simulink model "model"  (R2024a)
settings: Solver=VariableStepAuto  StartTime=0.0  StopTime=10  MaxStep=0.01  RelTol=1e-2
values from neighbouring files (symbols this model uses):
  K = lqr(A,B,Q,R)    [lqr_by_leg.m]    (also in setup.m = lqr_by_leg(0.218))
  N = NM + mp*diff(x + L*sin(theta),t,2)    [lqr_by_leg.m]
  T_max = 10    [setup.m]
  Tp_max = 100    [setup.m]
undefined symbols (not defined in the file or in its folder): X, Y, Z
libraries: sm_lib x86, nesl_utility x22, slpidlib x8
(part 4 of 4)

== matlab function model/forward_kinematics_virtual_speed1 ==
  data: d_phi0 output; phi_1 input; phi_4 input; d_phi1 input; d_phi4 input
function d_phi0 = fcn(phi_1,phi_4,d_phi1,d_phi4)
    L1 = 0.16;
    L2 = 0.196;
    L3 = 0.1959;
    L4 = 0.16;
    L5 = 0;
    
    d_phi0 = (d_phi1*((L1*cos(phi_1) + (2*L2*cos(2*atan(((4*L2^2*(L1*sin(phi_1) - L4*sin(phi_4))^2 - ((L1*sin(phi_1) - L4*sin(phi_4))^2 + (L5 - L1*cos(phi_1) + L4*cos(phi_4))^2 + L2^2 - L3^2)^2 + 4*L2^2*(L5 - L1*cos(phi_1) + L4*cos(phi_4))^2)^(1/2) - 2*L2*(L1*sin(phi_1) - L4*sin(phi_4)))/((L1*sin(phi_1) - L4*sin(phi_4))^2 + (L5 - L1*cos(phi_1) + L4*cos(phi_4))^2 + L2^2 - L3^2 + 2*L2*(L5 - L1*cos(phi_1) + L4*cos(phi_4)))))*(((8*L1*L2^2*cos(phi_1)*(L1*sin(phi_1) - L4*sin(phi_4)) - 2*(2*L1*cos(phi_1)*(L1*sin(phi_1) - L4*sin(phi_4)) + 2*L1*sin(phi_1)*(L5 - L1*cos(phi_1) + L4*cos(phi_4)))*((L1*sin(phi_1) - L4*sin(phi_4))^2 + (L5 - L1*cos(phi_1) + L4*cos(phi_4))^2 + L2^2 - L3^2) + 8*L1*L2^2*sin(phi_1)*(L5 - L1*cos(phi_1) + L4*cos(phi_4)))/(2*(4*L2^2*(L1*sin(phi_1) - L4*sin(phi_4))^2 - ((L1*sin(phi_1) - L4*sin(phi_4))^2 + (L5 - L1*cos(phi_1) + L4*cos(phi_4))^2 + L2^2 - L3^2)^2 + 4*L2^2*(L5 - L1*cos(phi_1) + L4*cos(phi_4))^2)^(1/2)) - 2*L1*L2*cos(phi_1))/((L1*sin(phi_1) - L4*sin(phi_4))^2 + (L5 - L1*cos(phi_1) + L4*cos(phi_4))^2 + L2^2 - L3^2 + 2*L2*(L5 - L1*cos(phi_1) + L4*cos(phi_4))) - (((4*L2^2*(L1*sin(phi_1) - L4*sin(phi_4))^2 - ((L1*sin(phi_1) - L4*sin(phi_4))^2 + (L5 - L1*cos(phi_1) + L4*cos(phi_4))^2 + L2^2 - L3^2)^2 + 4*L2^2*(L5 - L1*cos(phi_1) + L4*cos(phi_4))^2)^(1/2) - 2*L2*(L1*sin(phi_1) - L4*sin(phi_4)))*(2*L1*L2*sin(phi_1) + 2*L1*cos(phi_1)*(L1*sin(phi_1) - L4*sin(phi_4)) + 2*L1*sin(phi_1)*(L5 - L1*cos(phi_1) + L4*cos(phi_4))))/((L1*sin(phi_1) - L4*sin(phi_4))^2 + (L5 - L1*cos(phi_1) + L4*cos(phi_4))^2 + L2^2 - L3^2 + 2*L2*(L5 - L1*cos(phi_1) + L4*cos(phi_4)))^2))/(((4*L2^2*(L1*sin(phi_1) - L4*sin(phi_4))^2 - ((L1*sin(phi_1) - L4*sin(phi_4))^2 + (L5 - L1*cos(phi_1) + L4*cos(phi_4))^2 + L2^2 - L3^2)^2 + 4*L2^2*(L5 - L1*cos(phi_1) + L4*cos(phi_4))^2)^(1/2) - 2*L2*(L1*sin(phi_1) - L4*sin(phi_4)))^2/((L1*sin(phi_1) - L4*sin(phi_4))^2 + (L5 - L1*cos(phi_1) + L4*cos(phi_4))^2 + L2^2 - L3^2 + 2*L2*(L5 - L1*cos(phi_1) + L4*cos(phi_4)))^2 + 1))/(L2*cos(2*atan(((4*L2^2*(L1*sin(phi_1) - L4*sin(phi_4))^2 - ((L1*sin(phi_1) - L4*sin(phi_4))^2 + (L5 - L1*cos(phi_1) + L4*cos(phi_4))^2 + L2^2 - L3^2)^2 + 4*L2^2*(L5 - L1*cos(phi_1) + L4*cos(phi_4))^2)^(1/2) - 2*L2*(L1*sin(phi_1) - L4*sin(phi_4)))/((L1*sin(phi_1) - L4*sin(phi_4))^2 + (L5 - L1*cos(phi_1) + L4*cos(phi_4))^2 + L2^2 - L3^2 + 2*L2*(L5 - L1*cos(phi_1) + L4*cos(phi_4))))) - L5/2 + L1*cos(phi_1)) + ((L2*sin(2*atan(((4*L2^2*(L1*sin(phi_1) - L4*sin(phi_4))^2 - ((L1*sin(phi_1) - L4*sin(phi_4))^2 + (L5 - L1*cos(phi_1) + L4*cos(phi_4))^2 + L2^2 - L3^2)^2 + 4*L2^2*(L5 - L1*cos(phi_1) + L4*cos(phi_4))^2)^(1/2) - 2*L2*(L1*sin(phi_1) - L4*sin(phi_4)))/((L1*sin(phi_1) - L4*sin(phi_4))^2 + (L5 - L1*cos(phi_1) + L4*cos(phi_4))^2 + L2^2 - L3^2 + 2*L2*(L5 - L1*cos(phi_1) + L4*cos(phi_4))))) + L1*sin(phi_1))*(L1*sin(phi_1) + (2*L2*sin(2*atan(((4*L2^2*(L1*sin(phi_1) - L4*sin(phi_4))^2 - ((L1*sin(phi_1) - L4*sin(phi_4))^2 + (L5 - L1*cos(phi_1) + L4*cos(phi_4))^2 + L2^2 - L3^2)^2 + 4*L2^2*(L5 - L1*cos(phi_1) + L4*cos(phi_4))^2)^(1/2) - 2*L2*(L1*sin(phi_1) - L4*sin(phi_4)))/((L1*sin(phi_1) - L4*sin(phi_4))^2 + (L5 - L1*cos(phi_1) + L4*cos(phi_4))^2 + L2^2 - L3^2 + 2*L2*(L5 - L1*cos(phi_1) + L4*cos(phi_4)))))*(((8*L1*L2^2*cos(phi_1)*(L1*sin(phi_1) - L4*sin(phi_4)) - 2*(2*L1*cos(phi_1)*(L1*sin(phi_1) - L4*sin(phi_4)) + 2*L1*sin(phi_1)*(L5 - L1*cos(phi_1) + L4*cos(phi_4)))*((L1*sin(phi_1) - L4*sin(phi_4))^2 + (L5 - L1*cos(phi_1) + L4*cos(phi_4))^2 + L2^2 - L3^2) + 8*L1*L2^2*sin(phi_1)*(L5 - L1*cos(phi_1) + L4*cos(phi_4)))/(2*(4*L2^2*(L1*sin(phi_1) - L4*sin(phi_4))^2 - ((L1*sin(phi_1) - L4*sin(phi_4))^2 + (L5 - L1*cos(phi_1) + L4*cos(phi_4))^2 + L2^2 - L3^2)^2 + 4*L2^2*(L5 - L1*cos(phi_1) + L4*cos(phi_4))^2)^(1/2)) - 2*L1*L2*cos(phi_1))/((L1*sin(phi_1) - L4*sin(phi_4))^2 + (L5 - L1*cos(phi_1) + L4*cos(phi_4))^2 + L2^2 - L3^2 + 2*L2*(L5 - L1*cos(phi_1) + L4*cos(phi_4))) - (((4*L2^2*(L1*sin(phi_1) - L4*sin(phi_4))^2 - ((L1*sin(phi_1) - L4*sin(phi_4))^2 + (L5 - L1*cos(phi_1) + L4*cos(phi_4))^2 + L2^2 - L3^2)^2 + 4*L2^2*(L5 - L1*cos(phi_1) + L4*cos(phi_4))^2)^(1/2) - 2*L2*(L1*sin(phi_1) - L4*sin(phi_4)))*(2*L1*L2*sin(phi_1) + 2*L1*cos(phi_1)*(L1*sin(phi_1) - L4*sin(phi_4)) + 2*L1*sin(phi_1)*(L5 - L1*cos(phi_1) + L4*cos(phi_4))))/((L1*sin(phi_1) - L4*sin(phi_4))^2 + (L5 - L1*cos(phi_1) + L4*cos(phi_4))^2 + L2^2 - L3^2 + 2*L2*(L5 - L1*cos(phi_1) + L4*cos(phi_4)))^2))/(((4*L2^2*(L1*sin(phi_1) - L4*sin(phi_4))^2 - ((L1*sin(phi_1) - L4*sin(phi_4))^2 + (L5 - L1*cos(phi_1) + L4*cos(phi_4))^2 + L2^2 - L3^2)^2 + 4*L2^2*(L5 - L1*cos(phi_1) + L4*cos(phi_4))^2)^(1/2) - 2*L2*(L1*sin(phi_1) - L4*sin(phi_4)))^2/((L1*sin(phi_1) - L4*sin(phi_4))^2 + (L5 - L1*cos(phi_1) + L4*cos(phi_4))^2 + L2^2 - L3^2 + 2*L2*(L5 - L1*cos(phi_1) + L4*cos(phi_4)))^2 + 1)))/(L2*cos(2*atan(((4*L2^2*(L1*sin(phi_1) - L4*sin(phi_4))^2 - ((L1*sin(phi_1) - L4*sin(phi_4))^2 + (L5 - L1*cos(phi_1) + L4*cos(phi_4))^2 + L2^2 - L3^2)^2 + 4*L2^2*(L5 - L1*cos(phi_1) + L4*cos(phi_4))^2)^(1/2) - 2*L2*(L1*sin(phi_1) - L4*sin(phi_4)))/((L1*sin(phi_1) - L4*sin(phi_4))^2 + (L5 - L1*cos(phi_1) + L4*cos(phi_4))^2 + L2^2 - L3^2 + 2*L2*(L5 - L1*cos(phi_1) + L4*cos(phi_4))))) - L5/2 + L1*cos(phi_1))^2))/((L2*sin(2*atan(((4*L2^2*(L1*sin(phi_1) - L4*sin(phi_4))^2 - ((L1*sin(phi_1) - L4*sin(phi_4))^2 + (L5 - L1*cos(phi_1) + L4*cos(phi_4))^2 + L2^2 - L3^2)^2 + 4*L2^2*(L5 - L1*cos(phi_1) + L4*cos(phi_4))^2)^(1/2) - 2*L2*(L1*sin(phi_1) - L4*sin(phi_4)))/((L1*sin(phi_1) - L4*sin(phi_4))^2 + (L5 - L1*cos(phi_1) + L4*cos(phi_4))^2 + L2^2 - L3^2 + 2*L2*(L5 - L1*cos(phi_1) + L4*cos(phi_4))))) + L1*sin(phi_1))^2/(L2*cos(2*atan(((4*L2^2*(L1*sin(phi_1) - L4*sin(phi_4))^2 - ((L1*sin(phi_1) - L4*sin(phi_4))^2 + (L5 - L1*cos(phi_1) + L4*cos(phi_4))^2 + L2^2 - L3^2)^2 + 4*L2^2*(L5 - L1*cos(phi_1) + L4*cos(phi_4))^2)^(1/2) - 2*L2*(L1*sin(phi_1) - L4*sin(phi_4)))/((L1*sin(phi_1) - L4*sin(phi_4))^2 + (L5 - L1*cos(phi_1) + L4*cos(phi_4))^2 + L2^2 - L3^2 + 2*L2*(L5 - L1*cos(phi_1) + L4*cos(phi_4))))) - L5/2 + L1*cos(phi_1))^2 + 1) - (d_phi4*((2*L2*cos(2*atan(((4*L2^2*(L1*sin(phi_1) - L4*sin(phi_4))^2 - ((L1*sin(phi_1) - L4*sin(phi_4))^2 + (L5 - L1*cos(phi_1) + L4*cos(phi_4))^2 + L2^2 - L3^2)^2 + 4*L2^2*(L5 - L1*cos(phi_1) + L4*cos(phi_4))^2)^(1/2) - 2*L2*(L1*sin(phi_1) - L4*sin(phi_4)))/((L1*sin(phi_1) - L4*sin(phi_4))^2 + (L5 - L1*cos(phi_1) + L4*cos(phi_4))^2 + L2^2 - L3^2 + 2*L2*(L5 - L1*cos(phi_1) + L4*cos(phi_4)))))*(((8*L2^2*L4*cos(phi_4)*(L1*sin(phi_1) - L4*sin(phi_4)) - 2*(2*L4*cos(phi_4)*(L1*sin(phi_1) - L4*sin(phi_4)) + 2*L4*sin(phi_4)*(L5 - L1*cos(phi_1) + L4*cos(phi_4)))*((L1*sin(phi_1) - L4*sin(phi_4))^2 + (L5 - L1*cos(phi_1) + L4*cos(phi_4))^2 + L2^2 - L3^2) + 8*L2^2*L4*sin(phi_4)*(L5 - L1*cos(phi_1) + L4*cos(phi_4)))/(2*(4*L2^2*(L1*sin(phi_1) - L4*sin(phi_4))^2 - ((L1*sin(phi_1) - L4*sin(phi_4))^2 + (L5 - L1*cos(phi_1) + L4*cos(phi_4))^2 + L2^2 - L3^2)^2 + 4*L2^2*(L5 - L1*cos(phi_1) + L4*cos(phi_4))^2)^(1/2)) - 2*L2*L4*cos(phi_4))/((L1*sin(phi_1) - L4*sin(phi_4))^2 + (L5 - L1*cos(phi_1) + L4*cos(phi_4))^2 + L2^2 - L3^2 + 2*L2*(L5 - L1*cos(phi_1) + L4*cos(phi_4))) - (((4*L2^2*(L1*sin(phi_1) - L4*sin(phi_4))^2 - ((L1*sin(phi_1) - L4*sin(phi_4))^2 + (L5 - L1*cos(phi_1) + L4*cos(phi_4))^2 + L2^2 - L3^2)^2 + 4*L2^2*(L5 - L1*cos(phi_1) + L4*cos(phi_4))^2)^(1/2) - 2*L2*(L1*sin(phi_1) - L4*sin(phi_4)))*(2*L2*L4*sin(phi_4) + 2*L4*cos(phi_4)*(L1*sin(phi_1) - L4*sin(phi_4)) + 2*L4*sin(phi_4)*(L5 - L1*cos(phi_1) + L4*cos(phi_4))))/((L1*sin(phi_1) - L4*sin(phi_4))^2 + (L5 - L1*cos(phi_1) + L4*cos(phi_4))^2 + L2^2 - L3^2 + 2*L2*(L5 - L1*cos(phi_1) + L4*cos(phi_4)))^2))/((((4*L2^2*(L1*sin(phi_1) - L4*sin(phi_4))^2 - ((L1*sin(phi_1) - L4*sin(phi_4))^2 + (L5 - L1*cos(phi_1) + L4*cos(phi_4))^2 + L2^2 - L3^2)^2 + 4*L2^2*(L5 - L1*cos(phi_1) + L4*cos(phi_4))^2)^(1/2) - 2*L2*(L1*sin(phi_1) - L4*sin(phi_4)))^2/((L1*sin(phi_1) - L4*sin(phi_4))^2 + (L5 - L1*cos(phi_1) + L4*cos(phi_4))^2 + L2^2 - L3^2 + 2*L2*(L5 - L1*cos(phi_1) + L4*cos(phi_4)))^2 + 1)*(L2*cos(2*atan(((4*L2^2*(L1*sin(phi_1) - L4*sin(phi_4))^2 - ((L1*sin(phi_1) - L4*sin(phi_4))^2 + (L5 - L1*cos(phi_1) + L4*cos(phi_4))^2 + L2^2 - L3^2)^2 + 4*L2^2*(L5 - L1*cos(phi_1) + L4*cos(phi_4))^2)^(1/2) - 2*L2*(L1*sin(phi_1) - L4*sin(phi_4)))/((L1*sin(phi_1) - L4*sin(phi_4))^2 + (L5 - L1*cos(phi_1) + L4*cos(phi_4))^2 + L2^2 - L3^2 + 2*L2*(L5 - L1*cos(phi_1) + L4*cos(phi_4))))) - L5/2 + L1*cos(phi_1))) + (2*L2*sin(2*atan(((4*L2^2*(L1*sin(phi_1) - L4*sin(phi_4))^2 - ((L1*sin(phi_1) - L4*sin(phi_4))^2 + (L5 - L1*cos(phi_1) + L4*cos(phi_4))^2 + L2^2 - L3^2)^2 + 4*L2^2*(L5 - L1*cos(phi_1) + L4*cos(phi_4))^2)^(1/2) - 2*L2*(L1*sin(phi_1) - L4*sin(phi_4)))/((L1*sin(phi_1) - L4*sin(phi_4))^2 + (L5 - L1*cos(phi_1) + L4*cos(phi_4))^2 + L2^2 - L3^2 + 2*L2*(L5 - L1*cos(phi_1) + L4*cos(phi_4)))))*(L2*sin(2*atan(((4*L2^2*(L1*sin(phi_1) - L4*sin(phi_4))^2 - ((L1*sin(phi_1) - L4*sin(phi_4))^2 + (L5 - L1*cos(phi_1) + L4*cos(phi_4))^2 + L2^2 - L3^2)^2 + 4*L2^2*(L5 - L1*cos(phi_1) + L4*cos(phi_4))^2)^(1/2) - 2*L2*(L1*sin(phi_1) - L4*sin(phi_4)))/((L1*sin(phi_1) - L4*sin(phi_4))^2 + (L5 - L1*cos(phi_1) + L4*cos(phi_4))^2 + L2^2 - L3^2 + 2*L2*(L5 - L1*cos(phi_1) + L4*cos(phi_4))))) + L1*sin(phi_1))*(((8*L2^2*L4*cos(phi_4)*(L1*sin(phi_1) - L4*sin(phi_4)) - 2*(2*L4*cos(phi_4)*(L1*sin(phi_1) - L4*sin(phi_4)) + 2*L4*sin(phi_4)*(L5 - L1*cos(phi_1) + L4*cos(phi_4)))*((L1*sin(phi_1) - L4*sin(phi_4))^2 + (L5 - L1*cos(phi_1) + L4*cos(phi_4))^2 + L2^2 - L3^2) + 8*L2^2*L4*sin(phi_4)*(L5 - L1*cos(phi_1) + L4*cos(phi_4)))/(2*(4*L2^2*(L1*sin(phi_1) - L4*sin(phi_4))^2 - ((L1*sin(phi_1) - L4*sin(phi_4))^2 + (L5 - L1*cos(phi_1) + L4*cos(phi_4))^2 + L2^2 - L3^2)^2 + 4*L2^2*(L5 - L1*cos(phi_1) + L4*cos(phi_4))^2)^(1/2)) - 2*L2*L4*cos(phi_4))/((L1*sin(phi_1) - L4*sin(phi_4))^2 + (L5 - L1*cos(phi_1) + L4*cos(phi_4))^2 + L2^2 - L3^2 + 2*L2*(L5 - L1*cos(phi_1) + L4*cos(phi_4))) - (((4*L2^2*(L1*sin(phi_1) - L4*sin(phi_4))^2 - ((L1*sin(phi_1) - L4*sin(phi_4))^2 + (L5 - L1*cos(phi_1) + L4*cos(phi_4))^2 + L2^2 - L3^2)^2 + 4*L2^2*(L5 - L1*cos(phi_1) + L4*cos(phi_4))^2)^(1/2) - 2*L2*(L1*sin(phi_1) - L4*sin(phi_4)))*(2*L2*L4*sin(phi_4) + 2*L4*cos(phi_4)*(L1*sin(phi_1) - L4*sin(phi_4)) + 2*L4*sin(phi_4)*(L5 - L1*cos(phi_1) + L4*cos(phi_4))))/((L1*sin(phi_1) - L4*sin(phi_4))^2 + (L5 - L1*cos(phi_1) + L4*cos(phi_4))^2 + L2^2 - L3^2 + 2*L2*(L5 - L1*cos(phi_1) + L4*cos(phi_4)))^2))/((((4*L2^2*(L1*sin(phi_1) - L4*sin(phi_4))^2 - ((L1*sin(phi_1) - L4*sin(phi_4))^2 + (L5 - L1*cos(phi_1) + L4*cos(phi_4))^2 + L2^2 - L3^2)^2 + 4*L2^2*(L5 - L1*cos(phi_1) + L4*cos(phi_4))^2)^(1/2) - 2*L2*(L1*sin(phi_1) - L4*sin(phi_4)))^2/((L1*sin(phi_1) - L4*sin(phi_4))^2 + (L5 - L1*cos(phi_1) + L4*cos(phi_4))^2 + L2^2 - L3^2 + 2*L2*(L5 - L1*cos(phi_1) + L4*cos(phi_4)))^2 + 1)*(L2*cos(2*atan(((4*L2^2*(L1*sin(phi_1) - L4*sin(phi_4))^2 - ((L1*sin(phi_1) - L4*sin(phi_4))^2 + (L5 - L1*cos(phi_1) + L4*cos(phi_4))^2 + L2^2 - L3^2)^2 + 4*L2^2*(L5 - L1*cos(phi_1) + L4*cos(phi_4))^2)^(1/2) - 2*L2*(L1*sin(phi_1) - L4*sin(phi_4)))/((L1*sin(phi_1) - L4*sin(phi_4))^2 + (L5 - L1*cos(phi_1) + L4*cos(phi_4))^2 + L2^2 - L3^2 + 2*L2*(L5 - L1*cos(phi_1) + L4*cos(phi_4))))) - L5/2 + L1*cos(phi_1))^2)))/((L2*sin(2*atan(((4*L2^2*(L1*sin(phi_1) - L4*sin(phi_4))^2 - ((L1*sin(phi_1) - L4*sin(phi_4))^2 + (L5 - L1*cos(phi_1) + L4*cos(phi_4))^2 + L2^2 - L3^2)^2 + 4*L2^2*(L5 - L1*cos(phi_1) + L4*cos(phi_4))^2)^(1/2) - 2*L2*(L1*sin(phi_1) - L4*sin(phi_4)))/((L1*sin(phi_1) - L4*sin(phi_4))^2 + (L5 - L1*cos(phi_1) + L4*cos(phi_4))^2 + L2^2 - L3^2 + 2*L2*(L5 - L1*cos(phi_1) + L4*cos(phi_4))))) + L1*sin(phi_1))^2/(L2*cos(2*atan(((4*L2^2*(L1*sin(phi_1) - L4*sin(phi_4))^2 - ((L1*sin(phi_1) - L4*sin(phi_4))^2 + (L5 - L1*cos(phi_1) + L4*cos(phi_4))^2 + L2^2 - L3^2)^2 + 4*L2^2*(L5 - L1*cos(phi_1) + L4*cos(phi_4))^2)^(1/2) - 2*L2*(L1*sin(phi_1) - L4*sin(phi_4)))/((L1*sin(phi_1) - L4*sin(phi_4))^2 + (L5 - L1*cos(phi_1) + L4*cos(phi_4))^2 + L2^2 - L3^2 + 2*L2*(L5 - L1*cos(phi_1) + L4*cos(phi_4))))) - L5/2 + L1*cos(phi_1))^2 + 1);
end

    % syms phi_0 phi_1 phi_2 phi_4 L1 L2 L3 L4 L5 L0 d_phi1 d_phi4
    % 
    % XD=L5+L4*cos(phi_4);
    % YD=L4*sin(phi_4);
    % XB=L1*cos(phi_1);
    % YB=L1*sin(phi_1);
    % A0=2*L2*(XD-XB);
    % B0=2*L2*(YD-YB);
    % lBD=sqrt((XD-XB)^2+(YD-YB)^2);
    % C0=L2^2+lBD^2-L3^2;
    % phi_2=2*atan((B0+sqrt(A0^2+B0^2-C0^2))/(A0+C0));
    % XC=XB+L2*cos(phi_2);
    % YC=YB+L2*sin(phi_2);
    % L0=sqrt((XC-L5/2)^2+YC^2);
    % phi_0=atan(YC/(XC-L5/2));
    % 
    % J=jacobian([L0;phi_0],[phi_1;phi_4]);
    % phi0_dot = J(2,1)*d_phi1 +J(2,2)*d_phi4

    % jacobian函数无法在simulink中使用，故直接使用jacobian函数的最终结果

== matlab function model/MATLAB Function6 ==
  data: F0 input; T1 output; Tp input; phi1 input; phi4 input; T2 output
function [T1,T2] = VMC(F0,Tp,phi1,phi4)

    L5=0;%AE长度
    L1=0.16;
    L2=0.196;
    L3=0.196;
    L4=0.16;

    YD = L4*sin(phi4);
    YB = L1*sin(phi1);
    XD = L5 + L4*cos(phi4);
    XB = L1*cos(phi1); 
    lBD = sqrt((XD - XB)*(XD - XB) + (YD - YB)*(YD - YB));
    A0 = 2*L2*(XD - XB);
    B0 = 2*L2*(YD - YB);
    C0 = L2*L2 + lBD*lBD - L3*L3;
    phi2 = 2*atan2((B0 + sqrt(A0*A0 + B0*B0 - C0*C0)),A0 + C0);
    phi3 = atan2(YB-YD+L2*sin(phi2),XB-XD+L2*cos(phi2));
    XC = L1*cos(phi1) + L2*cos(phi2);
    YC = L1*sin(phi1) + L2*sin(phi2);
    L0 = sqrt((XC - L5/2)*(XC - L5/2) + YC*YC);
    phi0 = atan2(YC,XC - L5/2);
    j11 = (L1*sin(phi0-phi3)*sin(phi1-phi2))/sin(phi3-phi2);
    j12 = (L1*cos(phi0-phi3)*sin(phi1-phi2))/(L0*sin(phi3-phi2));
    j21 = (L4*sin(phi0-phi2)*sin(phi3-phi4))/sin(phi3-phi2);
    j22 = (L4*cos(phi0-phi2)*sin(phi3-phi4))/(L0*sin(phi3-phi2));
    J = [j11 j12; j21 j22];
    F = [F0;Tp];
    T = J * F;
    T1 = T(1,1);
    T2 = T(2,1);

end

== matlab function model/forward_kinematics_virtual_speed ==
  data: d_phi0 output; phi_1 input; phi_4 input; d_phi1 input; d_phi4 input
function d_phi0 = fcn(phi_1,phi_4,d_phi1,d_phi4)
    L1 = 0.16;
    L2 = 0.196;
    L3 = 0.1959;
    L4 = 0.16;
    L5=0;
    
    d_phi0 = (d_phi1*((L1*cos(phi_1) + (2*L2*cos(2*atan(((4*L2^2*(L1*sin(phi_1) - L4*sin(phi_4))^2 - ((L1*sin(phi_1) - L4*sin(phi_4))^2 + (L5 - L1*cos(phi_1) + L4*cos(phi_4))^2 + L2^2 - L3^2)^2 + 4*L2^2*(L5 - L1*cos(phi_1) + L4*cos(phi_4))^2)^(1/2) - 2*L2*(L1*sin(phi_1) - L4*sin(phi_4)))/((L1*sin(phi_1) - L4*sin(phi_4))^2 + (L5 - L1*cos(phi_1) + L4*cos(phi_4))^2 + L2^2 - L3^2 + 2*L2*(L5 - L1*cos(phi_1) + L4*cos(phi_4)))))*(((8*L1*L2^2*cos(phi_1)*(L1*sin(phi_1) - L4*sin(phi_4)) - 2*(2*L1*cos(phi_1)*(L1*sin(phi_1) - L4*sin(phi_4)) + 2*L1*sin(phi_1)*(L5 - L1*cos(phi_1) + L4*cos(phi_4)))*((L1*sin(phi_1) - L4*sin(phi_4))^2 + (L5 - L1*cos(phi_1) + L4*cos(phi_4))^2 + L2^2 - L3^2) + 8*L1*L2^2*sin(phi_1)*(L5 - L1*cos(phi_1) + L4*cos(phi_4)))/(2*(4*L2^2*(L1*sin(phi_1) - L4*sin(phi_4))^2 - ((L1*sin(phi_1) - L4*sin(phi_4))^2 + (L5 - L1*cos(phi_1) + L4*cos(phi_4))^2 + L2^2 - L3^2)^2 + 4*L2^2*(L5 - L1*cos(phi_1) + L4*cos(phi_4))^2)^(1/2)) - 2*L1*L2*cos(phi_1))/((L1*sin(phi_1) - L4*sin(phi_4))^2 + (L5 - L1*cos(phi_1) + L4*cos(phi_4))^2 + L2^2 - L3^2 + 2*L2*(L5 - L1*cos(phi_1) + L4*cos(phi_4))) - (((4*L2^2*(L1*sin(phi_1) - L4*sin(phi_4))^2 - ((L1*sin(phi_1) - L4*sin(phi_4))^2 + (L5 - L1*cos(phi_1) + L4*cos(phi_4))^2 + L2^2 - L3^2)^2 + 4*L2^2*(L5 - L1*cos(phi_1) + L4*cos(phi_4))^2)^(1/2) - 2*L2*(L1*sin(phi_1) - L4*sin(phi_4)))*(2*L1*L2*sin(phi_1) + 2*L1*cos(phi_1)*(L1*sin(phi_1) - L4*sin(phi_4)) + 2*L1*sin(phi_1)*(L5 - L1*cos(phi_1) + L4*cos(phi_4))))/((L1*sin(phi_1) - L4*sin(phi_4))^2 + (L5 - L1*cos(phi_1) + L4*cos(phi_4))^2 + L2^2 - L3^2 + 2*L2*(L5 - L1*cos(phi_1) + L4*cos(phi_4)))^2))/(((4*L2^2*(L1*sin(phi_1) - L4*sin(phi_4))^2 - ((L1*sin(phi_1) - L4*sin(phi_4))^2 + (L5 - L1*cos(phi_1) + L4*cos(phi_4))^2 + L2^2 - L3^2)^2 + 4*L2^2*(L5 - L1*cos(phi_1) + L4*cos(phi_4))^2)^(1/2) - 2*L2*(L1*sin(phi_1) - L4*sin(phi_4)))^2/((L1*sin(phi_1) - L4*sin(phi_4))^2 + (L5 - L1*cos(phi_1) + L4*cos(phi_4))^2 + L2^2 - L3^2 + 2*L2*(L5 - L1*cos(phi_1) + L4*cos(phi_4)))^2 + 1))/(L2*cos(2*atan(((4*L2^2*(L1*sin(phi_1) - L4*sin(phi_4))^2 - ((L1*sin(phi_1) - L4*sin(phi_4))^2 + (L5 - L1*cos(phi_1) + L4*cos(phi_4))^2 + L2^2 - L3^2)^2 + 4*L2^2*(L5 - L1*cos(phi_1) + L4*cos(phi_4))^2)^(1/2) - 2*L2*(L1*sin(phi_1) - L4*sin(phi_4)))/((L1*sin(phi_1) - L4*sin(phi_4))^2 + (L5 - L1*cos(phi_1) + L4*cos(phi_4))^2 + L2^2 - L3^2 + 2*L2*(L5 - L1*cos(phi_1) + L4*cos(phi_4))))) - L5/2 + L1*cos(phi_1)) + ((L2*sin(2*atan(((4*L2^2*(L1*sin(phi_1) - L4*sin(phi_4))^2 - ((L1*sin(phi_1) - L4*sin(phi_4))^2 + (L5 - L1*cos(phi_1) + L4*cos(phi_4))^2 + L2^2 - L3^2)^2 + 4*L2^2*(L5 - L1*cos(phi_1) + L4*cos(phi_4))^2)^(1/2) - 2*L2*(L1*sin(phi_1) - L4*sin(phi_4)))/((L1*sin(phi_1) - L4*sin(phi_4))^2 + (L5 - L1*cos(phi_1) + L4*cos(phi_4))^2 + L2^2 - L3^2 + 2*L2*(L5 - L1*cos(phi_1) + L4*cos(phi_4))))) + L1*sin(phi_1))*(L1*sin(phi_1) + (2*L2*sin(2*atan(((4*L2^2*(L1*sin(phi_1) - L4*sin(phi_4))^2 - ((L1*sin(phi_1) - L4*sin(phi_4))^2 + (L5 - L1*cos(phi_1) + L4*cos(phi_4))^2 + L2^2 - L3^2)^2 + 4*L2^2*(L5 - L1*cos(phi_1) + L4*cos(phi_4))^2)^(1/2) - 2*L2*(L1*sin(phi_1) - L4*sin(phi_4)))/((L1*sin(phi_1) - L4*sin(phi_4))^2 + (L5 - L1*cos(phi_1) + L4*cos(phi_4))^2 + L2^2 - L3^2 + 2*L2*(L5 - L1*cos(phi_1) + L4*cos(phi_4)))))*(((8*L1*L2^2*cos(phi_1)*(L1*sin(phi_1) - L4*sin(phi_4)) - 2*(2*L1*cos(phi_1)*(L1*sin(phi_1) - L4*sin(phi_4)) + 2*L1*sin(phi_1)*(L5 - L1*cos(phi_1) + L4*cos(phi_4)))*((L1*sin(phi_1) - L4*sin(phi_4))^2 + (L5 - L1*cos(phi_1) + L4*cos(phi_4))^2 + L2^2 - L3^2) + 8*L1*L2^2*sin(phi_1)*(L5 - L1*cos(phi_1) + L4*cos(phi_4)))/(2*(4*L2^2*(L1*sin(phi_1) - L4*sin(phi_4))^2 - ((L1*sin(phi_1) - L4*sin(phi_4))^2 + (L5 - L1*cos(phi_1) + L4*cos(phi_4))^2 + L2^2 - L3^2)^2 + 4*L2^2*(L5 - L1*cos(phi_1) + L4*cos(phi_4))^2)^(1/2)) - 2*L1*L2*cos(phi_1))/((L1*sin(phi_1) - L4*sin(phi_4))^2 + (L5 - L1*cos(phi_1) + L4*cos(phi_4))^2 + L2^2 - L3^2 + 2*L2*(L5 - L1*cos(phi_1) + L4*cos(phi_4))) - (((4*L2^2*(L1*sin(phi_1) - L4*sin(phi_4))^2 - ((L1*sin(phi_1) - L4*sin(phi_4))^2 + (L5 - L1*cos(phi_1) + L4*cos(phi_4))^2 + L2^2 - L3^2)^2 + 4*L2^2*(L5 - L1*cos(phi_1) + L4*cos(phi_4))^2)^(1/2) - 2*L2*(L1*sin(phi_1) - L4*sin(phi_4)))*(2*L1*L2*sin(phi_1) + 2*L1*cos(phi_1)*(L1*sin(phi_1) - L4*sin(phi_4)) + 2*L1*sin(phi_1)*(L5 - L1*cos(phi_1) + L4*cos(phi_4))))/((L1*sin(phi_1) - L4*sin(phi_4))^2 + (L5 - L1*cos(phi_1) + L4*cos(phi_4))^2 + L2^2 - L3^2 + 2*L2*(L5 - L1*cos(phi_1) + L4*cos(phi_4)))^2))/(((4*L2^2*(L1*sin(phi_1) - L4*sin(phi_4))^2 - ((L1*sin(phi_1) - L4*sin(phi_4))^2 + (L5 - L1*cos(phi_1) + L4*cos(phi_4))^2 + L2^2 - L3^2)^2 + 4*L2^2*(L5 - L1*cos(phi_1) + L4*cos(phi_4))^2)^(1/2) - 2*L2*(L1*sin(phi_1) - L4*sin(phi_4)))^2/((L1*sin(phi_1) - L4*sin(phi_4))^2 + (L5 - L1*cos(phi_1) + L4*cos(phi_4))^2 + L2^2 - L3^2 + 2*L2*(L5 - L1*cos(phi_1) + L4*cos(phi_4)))^2 + 1)))/(L2*cos(2*atan(((4*L2^2*(L1*sin(phi_1) - L4*sin(phi_4))^2 - ((L1*sin(phi_1) - L4*sin(phi_4))^2 + (L5 - L1*cos(phi_1) + L4*cos(phi_4))^2 + L2^2 - L3^2)^2 + 4*L2^2*(L5 - L1*cos(phi_1) + L4*cos(phi_4))^2)^(1/2) - 2*L2*(L1*sin(phi_1) - L4*sin(phi_4)))/((L1*sin(phi_1) - L4*sin(phi_4))^2 + (L5 - L1*cos(phi_1) + L4*cos(phi_4))^2 + L2^2 - L3^2 + 2*L2*(L5 - L1*cos(phi_1) + L4*cos(phi_4))))) - L5/2 + L1*cos(phi_1))^2))/((L2*sin(2*atan(((4*L2^2*(L1*sin(phi_1) - L4*sin(phi_4))^2 - ((L1*sin(phi_1) - L4*sin(phi_4))^2 + (L5 - L1*cos(phi_1) + L4*cos(phi_4))^2 + L2^2 - L3^2)^2 + 4*L2^2*(L5 - L1*cos(phi_1) + L4*cos(phi_4))^2)^(1/2) - 2*L2*(L1*sin(phi_1) - L4*sin(phi_4)))/((L1*sin(phi_1) - L4*sin(phi_4))^2 + (L5 - L1*cos(phi_1) + L4*cos(phi_4))^2 + L2^2 - L3^2 + 2*L2*(L5 - L1*cos(phi_1) + L4*cos(phi_4))))) + L1*sin(phi_1))^2/(L2*cos(2*atan(((4*L2^2*(L1*sin(phi_1) - L4*sin(phi_4))^2 - ((L1*sin(phi_1) - L4*sin(phi_4))^2 + (L5 - L1*cos(phi_1) + L4*cos(phi_4))^2 + L2^2 - L3^2)^2 + 4*L2^2*(L5 - L1*cos(phi_1) + L4*cos(phi_4))^2)^(1/2) - 2*L2*(L1*sin(phi_1) - L4*sin(phi_4)))/((L1*sin(phi_1) - L4*sin(phi_4))^2 + (L5 - L1*cos(phi_1) + L4*cos(phi_4))^2 + L2^2 - L3^2 + 2*L2*(L5 - L1*cos(phi_1) + L4*cos(phi_4))))) - L5/2 + L1*cos(phi_1))^2 + 1) - (d_phi4*((2*L2*cos(2*atan(((4*L2^2*(L1*sin(phi_1) - L4*sin(phi_4))^2 - ((L1*sin(phi_1) - L4*sin(phi_4))^2 + (L5 - L1*cos(phi_1) + L4*cos(phi_4))^2 + L2^2 - L3^2)^2 + 4*L2^2*(L5 - L1*cos(phi_1) + L4*cos(phi_4))^2)^(1/2) - 2*L2*(L1*sin(phi_1) - L4*sin(phi_4)))/((L1*sin(phi_1) - L4*sin(phi_4))^2 + (L5 - L1*cos(phi_1) + L4*cos(phi_4))^2 + L2^2 - L3^2 + 2*L2*(L5 - L1*cos(phi_1) + L4*cos(phi_4)))))*(((8*L2^2*L4*cos(phi_4)*(L1*sin(phi_1) - L4*sin(phi_4)) - 2*(2*L4*cos(phi_4)*(L1*sin(phi_1) - L4*sin(phi_4)) + 2*L4*sin(phi_4)*(L5 - L1*cos(phi_1) + L4*cos(phi_4)))*((L1*sin(phi_1) - L4*sin(phi_4))^2 + (L5 - L1*cos(phi_1) + L4*cos(phi_4))^2 + L2^2 - L3^2) + 8*L2^2*L4*sin(phi_4)*(L5 - L1*cos(phi_1) + L4*cos(phi_4)))/(2*(4*L2^2*(L1*sin(phi_1) - L4*sin(phi_4))^2 - ((L1*sin(phi_1) - L4*sin(phi_4))^2 + (L5 - L1*cos(phi_1) + L4*cos(phi_4))^2 + L2^2 - L3^2)^2 + 4*L2^2*(L5 - L1*cos(phi_1) + L4*cos(phi_4))^2)^(1/2)) - 2*L2*L4*cos(phi_4))/((L1*sin(phi_1) - L4*sin(phi_4))^2 + (L5 - L1*cos(phi_1) + L4*cos(phi_4))^2 + L2^2 - L3^2 + 2*L2*(L5 - L1*cos(phi_1) + L4*cos(phi_4))) - (((4*L2^2*(L1*sin(phi_1) - L4*sin(phi_4))^2 - ((L1*sin(phi_1) - L4*sin(phi_4))^2 + (L5 - L1*cos(phi_1) + L4*cos(phi_4))^2 + L2^2 - L3^2)^2 + 4*L2^2*(L5 - L1*cos(phi_1) + L4*cos(phi_4))^2)^(1/2) - 2*L2*(L1*sin(phi_1) - L4*sin(phi_4)))*(2*L2*L4*sin(phi_4) + 2*L4*cos(phi_4)*(L1*sin(phi_1) - L4*sin(phi_4)) + 2*L4*sin(phi_4)*(L5 - L1*cos(phi_1) + L4*cos(phi_4))))/((L1*sin(phi_1) - L4*sin(phi_4))^2 + (L5 - L1*cos(phi_1) + L4*cos(phi_4))^2 + L2^2 - L3^2 + 2*L2*(L5 - L1*cos(phi_1) + L4*cos(phi_4)))^2))/((((4*L2^2*(L1*sin(phi_1) - L4*sin(phi_4))^2 - ((L1*sin(phi_1) - L4*sin(phi_4))^2 + (L5 - L1*cos(phi_1) + L4*cos(phi_4))^2 + L2^2 - L3^2)^2 + 4*L2^2*(L5 - L1*cos(phi_1) + L4*cos(phi_4))^2)^(1/2) - 2*L2*(L1*sin(phi_1) - L4*sin(phi_4)))^2/((L1*sin(phi_1) - L4*sin(phi_4))^2 + (L5 - L1*cos(phi_1) + L4*cos(phi_4))^2 + L2^2 - L3^2 + 2*L2*(L5 - L1*cos(phi_1) + L4*cos(phi_4)))^2 + 1)*(L2*cos(2*atan(((4*L2^2*(L1*sin(phi_1) - L4*sin(phi_4))^2 - ((L1*sin(phi_1) - L4*sin(phi_4))^2 + (L5 - L1*cos(phi_1) + L4*cos(phi_4))^2 + L2^2 - L3^2)^2 + 4*L2^2*(L5 - L1*cos(phi_1) + L4*cos(phi_4))^2)^(1/2) - 2*L2*(L1*sin(phi_1) - L4*sin(phi_4)))/((L1*sin(phi_1) - L4*sin(phi_4))^2 + (L5 - L1*cos(phi_1) + L4*cos(phi_4))^2 + L2^2 - L3^2 + 2*L2*(L5 - L1*cos(phi_1) + L4*cos(phi_4))))) - L5/2 + L1*cos(phi_1))) + (2*L2*sin(2*atan(((4*L2^2*(L1*sin(phi_1) - L4*sin(phi_4))^2 - ((L1*sin(phi_1) - L4*sin(phi_4))^2 + (L5 - L1*cos(phi_1) + L4*cos(phi_4))^2 + L2^2 - L3^2)^2 + 4*L2^2*(L5 - L1*cos(phi_1) + L4*cos(phi_4))^2)^(1/2) - 2*L2*(L1*sin(phi_1) - L4*sin(phi_4)))/((L1*sin(phi_1) - L4*sin(phi_4))^2 + (L5 - L1*cos(phi_1) + L4*cos(phi_4))^2 + L2^2 - L3^2 + 2*L2*(L5 - L1*cos(phi_1) + L4*cos(phi_4)))))*(L2*sin(2*atan(((4*L2^2*(L1*sin(phi_1) - L4*sin(phi_4))^2 - ((L1*sin(phi_1) - L4*sin(phi_4))^2 + (L5 - L1*cos(phi_1) + L4*cos(phi_4))^2 + L2^2 - L3^2)^2 + 4*L2^2*(L5 - L1*cos(phi_1) + L4*cos(phi_4))^2)^(1/2) - 2*L2*(L1*sin(phi_1) - L4*sin(phi_4)))/((L1*sin(phi_1) - L4*sin(phi_4))^2 + (L5 - L1*cos(phi_1) + L4*cos(phi_4))^2 + L2^2 - L3^2 + 2*L2*(L5 - L1*cos(phi_1) + L4*cos(phi_4))))) + L1*sin(phi_1))*(((8*L2^2*L4*cos(phi_4)*(L1*sin(phi_1) - L4*sin(phi_4)) - 2*(2*L4*cos(phi_4)*(L1*sin(phi_1) - L4*sin(phi_4)) + 2*L4*sin(phi_4)*(L5 - L1*cos(phi_1) + L4*cos(phi_4)))*((L1*sin(phi_1) - L4*sin(phi_4))^2 + (L5 - L1*cos(phi_1) + L4*cos(phi_4))^2 + L2^2 - L3^2) + 8*L2^2*L4*sin(phi_4)*(L5 - L1*cos(phi_1) + L4*cos(phi_4)))/(2*(4*L2^2*(L1*sin(phi_1) - L4*sin(phi_4))^2 - ((L1*sin(phi_1) - L4*sin(phi_4))^2 + (L5 - L1*cos(phi_1) + L4*cos(phi_4))^2 + L2^2 - L3^2)^2 + 4*L2^2*(L5 - L1*cos(phi_1) + L4*cos(phi_4))^2)^(1/2)) - 2*L2*L4*cos(phi_4))/((L1*sin(phi_1) - L4*sin(phi_4))^2 + (L5 - L1*cos(phi_1) + L4*cos(phi_4))^2 + L2^2 - L3^2 + 2*L2*(L5 - L1*cos(phi_1) + L4*cos(phi_4))) - (((4*L2^2*(L1*sin(phi_1) - L4*sin(phi_4))^2 - ((L1*sin(phi_1) - L4*sin(phi_4))^2 + (L5 - L1*cos(phi_1) + L4*cos(phi_4))^2 + L2^2 - L3^2)^2 + 4*L2^2*(L5 - L1*cos(phi_1) + L4*cos(phi_4))^2)^(1/2) - 2*L2*(L1*sin(phi_1) - L4*sin(phi_4)))*(2*L2*L4*sin(phi_4) + 2*L4*cos(phi_4)*(L1*sin(phi_1) - L4*sin(phi_4)) + 2*L4*sin(phi_4)*(L5 - L1*cos(phi_1) + L4*cos(phi_4))))/((L1*sin(phi_1) - L4*sin(phi_4))^2 + (L5 - L1*cos(phi_1) + L4*cos(phi_4))^2 + L2^2 - L3^2 + 2*L2*(L5 - L1*cos(phi_1) + L4*cos(phi_4)))^2))/((((4*L2^2*(L1*sin(phi_1) - L4*sin(phi_4))^2 - ((L1*sin(phi_1) - L4*sin(phi_4))^2 + (L5 - L1*cos(phi_1) + L4*cos(phi_4))^2 + L2^2 - L3^2)^2 + 4*L2^2*(L5 - L1*cos(phi_1) + L4*cos(phi_4))^2)^(1/2) - 2*L2*(L1*sin(phi_1) - L4*sin(phi_4)))^2/((L1*sin(phi_1) - L4*sin(phi_4))^2 + (L5 - L1*cos(phi_1) + L4*cos(phi_4))^2 + L2^2 - L3^2 + 2*L2*(L5 - L1*cos(phi_1) + L4*cos(phi_4)))^2 + 1)*(L2*cos(2*atan(((4*L2^2*(L1*sin(phi_1) - L4*sin(phi_4))^2 - ((L1*sin(phi_1) - L4*sin(phi_4))^2 + (L5 - L1*cos(phi_1) + L4*cos(phi_4))^2 + L2^2 - L3^2)^2 + 4*L2^2*(L5 - L1*cos(phi_1) + L4*cos(phi_4))^2)^(1/2) - 2*L2*(L1*sin(phi_1) - L4*sin(phi_4)))/((L1*sin(phi_1) - L4*sin(phi_4))^2 + (L5 - L1*cos(phi_1) + L4*cos(phi_4))^2 + L2^2 - L3^2 + 2*L2*(L5 - L1*cos(phi_1) + L4*cos(phi_4))))) - L5/2 + L1*cos(phi_1))^2)))/((L2*sin(2*atan(((4*L2^2*(L1*sin(phi_1) - L4*sin(phi_4))^2 - ((L1*sin(phi_1) - L4*sin(phi_4))^2 + (L5 - L1*cos(phi_1) + L4*cos(phi_4))^2 + L2^2 - L3^2)^2 + 4*L2^2*(L5 - L1*cos(phi_1) + L4*cos(phi_4))^2)^(1/2) - 2*L2*(L1*sin(phi_1) - L4*sin(phi_4)))/((L1*sin(phi_1) - L4*sin(phi_4))^2 + (L5 - L1*cos(phi_1) + L4*cos(phi_4))^2 + L2^2 - L3^2 + 2*L2*(L5 - L1*cos(phi_1) + L4*cos(phi_4))))) + L1*sin(phi_1))^2/(L2*cos(2*atan(((4*L2^2*(L1*sin(phi_1) - L4*sin(phi_4))^2 - ((L1*sin(phi_1) - L4*sin(phi_4))^2 + (L5 - L1*cos(phi_1) + L4*cos(phi_4))^2 + L2^2 - L3^2)^2 + 4*L2^2*(L5 - L1*cos(phi_1) + L4*cos(phi_4))^2)^(1/2) - 2*L2*(L1*sin(phi_1) - L4*sin(phi_4)))/((L1*sin(phi_1) - L4*sin(phi_4))^2 + (L5 - L1*cos(phi_1) + L4*cos(phi_4))^2 + L2^2 - L3^2 + 2*L2*(L5 - L1*cos(phi_1) + L4*cos(phi_4))))) - L5/2 + L1*cos(phi_1))^2 + 1);
end

    % syms phi_0 phi_1 phi_2 phi_4 L1 L2 L3 L4 L5 L0 d_phi1 d_phi4
    % 
    % XD=L5+L4*cos(phi_4);
    % YD=L4*sin(phi_4);
    % XB=L1*cos(phi_1);
    % YB=L1*sin(phi_1);
    % A0=2*L2*(XD-XB);
    % B0=2*L2*(YD-YB);
    % lBD=sqrt((XD-XB)^2+(YD-YB)^2);
    % C0=L2^2+lBD^2-L3^2;
    % phi_2=2*atan((B0+sqrt(A0^2+B0^2-C0^2))/(A0+C0));
    % XC=XB+L2*cos(phi_2);
    % YC=YB+L2*sin(phi_2);
    % L0=sqrt((XC-L5/2)^2+YC^2);
    % phi_0=atan(YC/(XC-L5/2));
    % 
    % J=jacobian([L0;phi_0],[phi_1;phi_4]);
    % phi0_dot = J(2,1)*d_phi1 +J(2,2)*d_phi4

    % jacobian函数无法在simulink中使用，故直接使用jacobian函数的最终结果
